simulink model "loopFilter_test"  (R2016b)
settings: Solver=VariableStepAuto  StartTime=0.0  StopTime=2^16/Fadc  RelTol=1e-3  EnableMultiTasking=on
PreLoadFcn:
  | setup
values from neighbouring files (symbols this model uses):
  Fadc = 614.4e6    (= 614400000)    [setup.m]
libraries: xbsIndex_r4 x13, simulink x1, CryoDetLibCMB x1
settings Model: Creator=Mitch  LastModifiedBy=mdewart
settings OptimizationCC: LifeSpan=inf
settings DebuggingCC: SFUnexpectedBacktrackingDiag=warning  SFNoUnconditionalDefaultTransitionDiag=warning  SFExecutionAtInitializationDiag=none
settings GRTTargetCC: TargetLangStandard=C89/C90 (ANSI)  GeneratePreprocessorConditionals=Disable all
settings ConfigComp: CovMetricSettings=dw  CovHtmlReporting=on  CovSaveCumulativeToWorkspaceVar=on  CovSaveSingleToWorkspaceVar=on  CovExternalEMLEnable=off

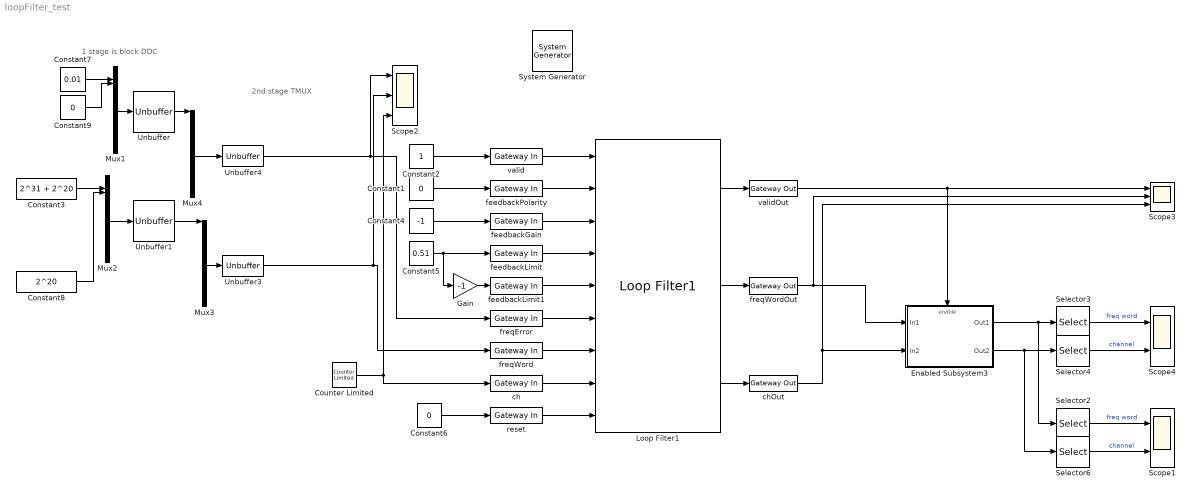
== system loopFilter_test ==
  note: 2nd stage TMUX
  note: 1 stage is block DDC
  " System Generator" : xbsIndex_r4/ System Generator  Tag=genX  xilinxfamily=kintexu  part=xcku040  speed=-2-e  package=ffva1156  synthesis_tool=Vivado  clock_wrapper=Clock Enables  directory=./netlist  proj_type=Vivado  Synth_file=Vivado Synthesis Defaults  Impl_file=Vivado Implementation Defaults  testbench=off  simulink_period=2/Fadc  sysclk_period=2e9/Fadc  dcm_input_clock_period=10  incr_netlist=off  trim_vbits=Everywhere in SubSystem  dbl_ovrd=According to Block Masks  core_generation=According to Block Masks  run_coregen=off  deprecated_control=off  eval_field=0  block_type=sysgen
  Constant1 : Constant  Value=0  SampleTime=2/Fadc
  Constant2 : Constant  SampleTime=2/Fadc
  Constant3 : Constant  Value=2^31 + 2^20  SampleTime=256/Fadc
  Constant4 : Constant  Value=-1  SampleTime=2/Fadc
  Constant5 : Constant  Value=0.51  SampleTime=2/Fadc
  Constant6 : Constant  Value=0  SampleTime=2/Fadc
  Constant7 : Constant  Value=0.01  SampleTime=256/Fadc
  Constant8 : Constant  Value=2^20  SampleTime=256/Fadc
  Constant9 : Constant  Value=0  SampleTime=256/Fadc
  Counter Limited : simulink/Sources/Counter Limited  uplimit=127  tsamp=2/Fadc
  Enabled Subsystem3 : Subsystem  TreatAsAtomicUnit=on
  Gain : Gain  Gain=-1
  Loop Filter1 : CryoDetLibCMB/Loop Filter1
  Mux1 : Mux  Inputs=16
  Mux2 : Mux  Inputs=16
  Mux3 : Mux  Inputs=8
  Mux4 : Mux  Inputs=8
  Scope1 : Scope  NumInputPorts=2
  Scope2 : Scope  NumInputPorts=3
  Scope3 : Scope  NumInputPorts=3
  Scope4 : Scope  NumInputPorts=2
  Selector2 : Selector  InputPortWidth=128  IndexOptions=Index vector (dialog)  Indices=[8+1]  OutputSizes=1
  Selector3 : Selector  InputPortWidth=128  IndexOptions=Index vector (dialog)  Indices=[1]  OutputSizes=1
  Selector4 : Selector  InputPortWidth=128  IndexOptions=Index vector (dialog)  Indices=[1]  OutputSizes=1
  Selector6 : Selector  InputPortWidth=128  IndexOptions=Index vector (dialog)  Indices=[8+1]  OutputSizes=1
  Unbuffer{,1,3..4} (4 alike) : Unbuffer  SampleBasedProcessing=Same as frame based
  ch : xbsIndex_r4/Gateway In  gui_display_data_type=Fixed-point  arith_type=Unsigned  n_bits=7  bin_pt=0  preci_type=Single  exp_width=8  frac_width=24  rows=1  columns=1  quantization="Round  (unbiased: +/- Inf)"  overflow=Saturate  period=2/Fadc  UseAsADC=off  ADCChannel='1'  interface=None  automatic_assignment=on  address_offset=hex2dec('00')  intf_name=''  intf_description=''  default_value=0  timing_constraint=None  locs_specified=off  LOCs={}  io_standard={}  inherit_from_input=off  hdl_port=on  dbl_ovrd=off  block_type=gatewayin
  chOut : xbsIndex_r4/Gateway Out  inherit_from_input=off  hdl_port=on  rows=1  columns=1  UseAsDAC=off  DACChannel='1'  interface=None  automatic_assignment=on  address_offset=hex2dec('00')  intf_name=''  intf_description=''  timing_constraint=None  locs_specified=off  LOCs={}  io_standard={}  block_type=gatewayout
  feedbackGain : xbsIndex_r4/Gateway In  gui_display_data_type=Fixed-point  arith_type="Signed  (2's comp)"  n_bits=16  bin_pt=14  preci_type=Single  exp_width=8  frac_width=24  rows=1  columns=1  quantization="Round  (unbiased: +/- Inf)"  overflow=Saturate  period=2/Fadc  UseAsADC=off  ADCChannel='1'  interface=None  automatic_assignment=on  address_offset=hex2dec('00')  intf_name=''  intf_description=''  default_value=0  timing_constraint=None  locs_specified=off  LOCs={}  io_standard={}  inherit_from_input=off  hdl_port=on  dbl_ovrd=off  block_type=gatewayin
  feedbackLimit : xbsIndex_r4/Gateway In  gui_display_data_type=Fixed-point  arith_type="Signed  (2's comp)"  n_bits=16  bin_pt=15  preci_type=Single  exp_width=8  frac_width=24  rows=1  columns=1  quantization="Round  (unbiased: +/- Inf)"  overflow=Saturate  period=2/Fadc  UseAsADC=off  ADCChannel='1'  interface=None  automatic_assignment=on  address_offset=hex2dec('00')  intf_name=''  intf_description=''  default_value=0  timing_constraint=None  locs_specified=off  LOCs={}  io_standard={}  inherit_from_input=off  hdl_port=on  dbl_ovrd=off  block_type=gatewayin
  feedbackLimit1 : xbsIndex_r4/Gateway In  gui_display_data_type=Fixed-point  arith_type="Signed  (2's comp)"  n_bits=16  bin_pt=15  preci_type=Single  exp_width=8  frac_width=24  rows=1  columns=1  quantization="Round  (unbiased: +/- Inf)"  overflow=Saturate  period=2/Fadc  UseAsADC=off  ADCChannel='1'  interface=None  automatic_assignment=on  address_offset=hex2dec('00')  intf_name=''  intf_description=''  default_value=0  timing_constraint=None  locs_specified=off  LOCs={}  io_standard={}  inherit_from_input=off  hdl_port=on  dbl_ovrd=off  block_type=gatewayin
  feedbackPolarity : xbsIndex_r4/Gateway In  gui_display_data_type=Fixed-point  arith_type=Unsigned  n_bits=1  bin_pt=0  preci_type=Single  exp_width=8  frac_width=24  rows=1  columns=1  quantization="Round  (unbiased: +/- Inf)"  overflow=Saturate  period=2/Fadc  UseAsADC=off  ADCChannel='1'  interface=None  automatic_assignment=on  address_offset=hex2dec('00')  intf_name=''  intf_description=''  default_value=0  timing_constraint=None  locs_specified=off  LOCs={}  io_standard={}  inherit_from_input=off  hdl_port=on  dbl_ovrd=off  block_type=gatewayin
  freqError : xbsIndex_r4/Gateway In  gui_display_data_type=Fixed-point  arith_type="Signed  (2's comp)"  n_bits=24  bin_pt=23  preci_type=Single  exp_width=8  frac_width=24  rows=1  columns=1  quantization="Round  (unbiased: +/- Inf)"  overflow=Wrap  period=2/Fadc  UseAsADC=off  ADCChannel='1'  interface=None  automatic_assignment=on  address_offset=hex2dec('00')  intf_name=''  intf_description=''  default_value=0  timing_constraint=None  locs_specified=off  LOCs={}  io_standard={}  inherit_from_input=off  hdl_port=on  dbl_ovrd=off  block_type=gatewayin
  freqWord : xbsIndex_r4/Gateway In  gui_display_data_type=Fixed-point  arith_type=Unsigned  n_bits=32  bin_pt=0  preci_type=Single  exp_width=8  frac_width=24  rows=1  columns=1  quantization="Round  (unbiased: +/- Inf)"  overflow=Saturate  period=2/Fadc  UseAsADC=off  ADCChannel='1'  interface=None  automatic_assignment=on  address_offset=hex2dec('00')  intf_name=''  intf_description=''  default_value=0  timing_constraint=None  locs_specified=off  LOCs={}  io_standard={}  inherit_from_input=off  hdl_port=on  dbl_ovrd=off  block_type=gatewayin
  freqWordOut : xbsIndex_r4/Gateway Out  inherit_from_input=off  hdl_port=on  rows=1  columns=1  UseAsDAC=off  DACChannel='1'  interface=None  automatic_assignment=on  address_offset=hex2dec('00')  intf_name=''  intf_description=''  timing_constraint=None  locs_specified=off  LOCs={}  io_standard={}  block_type=gatewayout
  reset : xbsIndex_r4/Gateway In  gui_display_data_type=Fixed-point  arith_type=Unsigned  n_bits=1  bin_pt=0  preci_type=Single  exp_width=8  frac_width=24  rows=1  columns=1  quantization="Round  (unbiased: +/- Inf)"  overflow=Saturate  period=2/Fadc  UseAsADC=off  ADCChannel='1'  interface=None  automatic_assignment=on  address_offset=hex2dec('00')  intf_name=''  intf_description=''  default_value=0  timing_constraint=None  locs_specified=off  LOCs={}  io_standard={}  inherit_from_input=off  hdl_port=on  dbl_ovrd=off  block_type=gatewayin
  valid : xbsIndex_r4/Gateway In  gui_display_data_type=Boolean  arith_type=Boolean  n_bits=18  bin_pt=15  preci_type=Single  exp_width=8  frac_width=24  rows=1  columns=1  quantization="Round  (unbiased: +/- Inf)"  overflow=Saturate  period=2/Fadc  UseAsADC=off  ADCChannel='1'  interface=None  automatic_assignment=on  address_offset=hex2dec('00')  intf_name=''  intf_description=''  default_value=0  timing_constraint=None  locs_specified=off  LOCs={}  io_standard={}  inherit_from_input=off  hdl_port=on  dbl_ovrd=off  block_type=gatewayin
  validOut : xbsIndex_r4/Gateway Out  inherit_from_input=off  hdl_port=on  rows=1  columns=1  UseAsDAC=off  DACChannel='1'  interface=None  automatic_assignment=on  address_offset=hex2dec('00')  intf_name=''  intf_description=''  timing_constraint=None  locs_specified=off  LOCs={}  io_standard={}  block_type=gatewayout
  wires:
  Constant2/1 -> valid/1
  Counter Limited/1 -> Scope2/3, ch/1
  Mux1/1 -> Unbuffer/1
  Unbuffer4/1 -> Scope2/1, freqError/1
  Loop Filter1/1 -> validOut/1
  Loop Filter1/2 -> freqWordOut/1
  Enabled Subsystem3/2(Out2) -> Selector6/1, Selector4/1
  Selector3/1 -> Scope4/1  "freq word"
  Selector4/1 -> Scope4/2  "channel"
  Constant1/1 -> feedbackPolarity/1
  Constant4/1 -> feedbackGain/1
  Constant5/1 -> Gain/1, feedbackLimit/1
  Constant6/1 -> reset/1
  Constant7/1 -> Mux1/1
  Mux2/1 -> Unbuffer1/1
  Unbuffer3/1 -> Scope2/2, freqWord/1
  Constant8/1 -> Mux2/2
  Constant9/1 -> Mux1/2
  Mux3/1 -> Unbuffer3/1
  Constant3/1 -> Mux2/1
  valid/1 -> Loop Filter1/1
  feedbackPolarity/1 -> Loop Filter1/2
  feedbackGain/1 -> Loop Filter1/3
  feedbackLimit/1 -> Loop Filter1/4
  reset/1 -> Loop Filter1/9
  ch/1 -> Loop Filter1/8
  Mux4/1 -> Unbuffer4/1
  freqWord/1 -> Loop Filter1/7
  freqError/1 -> Loop Filter1/6
  Loop Filter1/3 -> chOut/1
  validOut/1 -> Enabled Subsystem3/Enable, Scope3/1
  freqWordOut/1 -> Scope3/2, Enabled Subsystem3/1(In1)
  chOut/1 -> Enabled Subsystem3/2(In2), Scope3/3
  Selector2/1 -> Scope1/1  "freq word"
  Selector6/1 -> Scope1/2  "channel"
  Enabled Subsystem3/1(Out1) -> Selector2/1, Selector3/1
  Unbuffer/1 -> Mux4/1
  Unbuffer1/1 -> Mux3/1
  feedbackLimit1/1 -> Loop Filter1/5
  Gain/1 -> feedbackLimit1/1

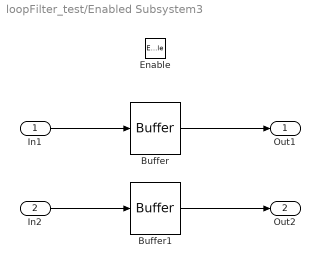
== system loopFilter_test/Enabled Subsystem3 ==
  In1 : Inport
  In2 : Inport  Port=2
  Enable : EnablePort
  Buffer : Buffer  N=128  TreatMby1Signals=One channel  OutputFrames=off
  Buffer1 : Buffer  N=128  TreatMby1Signals=One channel  OutputFrames=off
  Out1 : Outport
  Out2 : Outport  Port=2
  wires:
  In1/1 -> Buffer/1
  Buffer/1 -> Out1/1
  In2/1 -> Buffer1/1
  Buffer1/1 -> Out2/1
